simulink model "NAVI_V1"  (R2018a)
settings: configuration reference "Config_Ctrl" (kept outside this file)
PreLoadFcn:
  | NAVI_V1_BusInfo;
libraries: simulink x2
settings Model: Creator=IAEC nishito  LastModifiedBy=E00026
settings ConfigSetRef: SourceLocation=Base Workspace

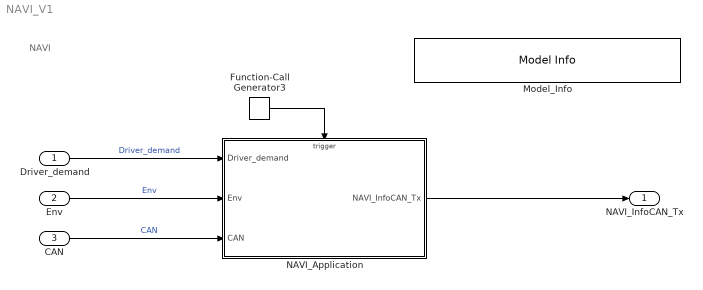
== system NAVI_V1 ==
  note: NAVI
  Driver_demand : Inport  OutDataTypeStr=Bus: Driver_demand_Bus
      settings: AttributesFormatString=<%<OutDataTypeStr>>
  Env : Inport  Port=2  OutDataTypeStr=Bus: Environment_Bus
      settings: AttributesFormatString=<%<OutDataTypeStr>>
  CAN : Inport  Port=3  OutDataTypeStr=Bus: CAN_Bus
      settings: AttributesFormatString=<%<OutDataTypeStr>>
  Function-Call Generator3 : simulink/Ports & Subsystems/Function-Call Generator  sample_time=0.1  numberOfIterations=1
      settings: AttributesFormatString=<sample_time=%<sample_time>>
  Model_Info : simulink/Model-Wide Utilities/Model Info  Frame=on  DisplayStringWithTags=|  HorizontalTextAlignment=Left  LeftAlignmentValue=0.02
      | Version  %<ModelVersion>
      | LastModifided by %<LastModifiedBy>  Date %<LastModificationDate>
      | Description  %<Description>
  NAVI_Application : Subsystem
  NAVI_InfoCAN_Tx : Outport  OutDataTypeStr=Bus: NAVI_InfoCAN_Tx_Bus
      settings: AttributesFormatString=<%<OutDataTypeStr>>
  wires:
  NAVI_Application/1(NAVI_InfoCAN_Tx) -> NAVI_InfoCAN_Tx/1
  CAN/1 -> NAVI_Application/3(CAN)  "CAN"
  Driver_demand/1 -> NAVI_Application/1(Driver_demand)  "Driver_demand"
  Function-Call Generator3/1 -> NAVI_Application/Trigger
  Env/1 -> NAVI_Application/2(Env)  "Env"

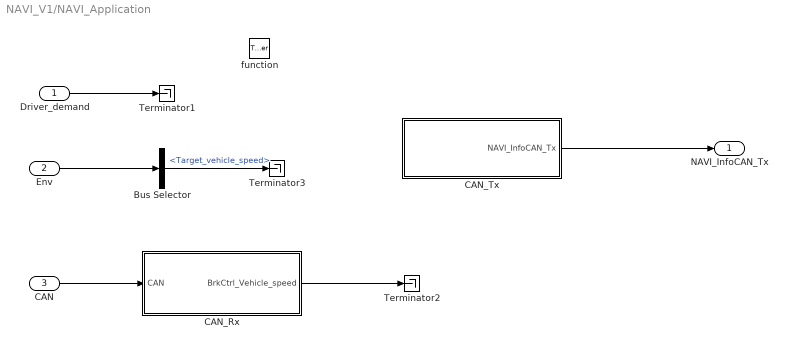
== system NAVI_V1/NAVI_Application ==
  Driver_demand : Inport
  Env : Inport  Port=2
  CAN : Inport  Port=3
  function : TriggerPort  TriggerType=function-call  VariantControl=Variant
  Bus Selector : BusSelector  OutputSignals=Target_vehicle_speed
  CAN_Rx : Subsystem
  CAN_Tx : Subsystem
  Terminator1 : Terminator
  Terminator2 : Terminator
  Terminator3 : Terminator
  NAVI_InfoCAN_Tx : Outport
  wires:
  Driver_demand/1 -> Terminator1/1
  CAN/1 -> CAN_Rx/1(CAN)
  CAN_Rx/1(BrkCtrl_Vehicle_speed) -> Terminator2/1
  Env/1 -> Bus Selector/1
  Bus Selector/1 -> Terminator3/1  "<Target_vehicle_speed>"
  CAN_Tx/1(NAVI_InfoCAN_Tx) -> NAVI_InfoCAN_Tx/1

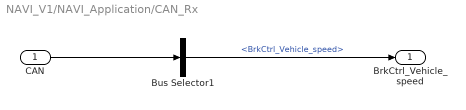
== system NAVI_V1/NAVI_Application/CAN_Rx ==
  CAN : Inport
  Bus Selector1 : BusSelector  OutputSignals=VehCAN.BrakeCtrl_VehCAN_Tx.BrkCtrl_Vehicle_speed
  BrkCtrl_Vehicle_speed : Outport
  wires:
  CAN/1 -> Bus Selector1/1
  Bus Selector1/1 -> BrkCtrl_Vehicle_speed/1  "<BrkCtrl_Vehicle_speed>"

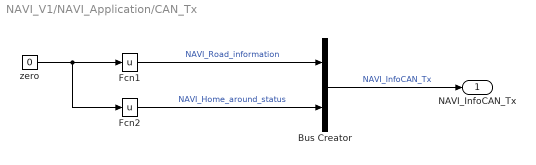
== system NAVI_V1/NAVI_Application/CAN_Tx ==
  Bus Creator : BusCreator  Inputs=2  OutDataTypeStr=Bus: NAVI_InfoCAN_Tx_Bus
      settings: AttributesFormatString=<%<OutDataTypeStr>>
  Fcn1 : Fcn  Expr=u
  Fcn2 : Fcn  Expr=u
  zero : Constant  Value=0
  NAVI_InfoCAN_Tx : Outport
  wires:
  Fcn1/1 -> Bus Creator/1  "NAVI_Road_information"
  zero/1 -> Fcn1/1, Fcn2/1
  Fcn2/1 -> Bus Creator/2  "NAVI_Home_around_status"
  Bus Creator/1 -> NAVI_InfoCAN_Tx/1  "NAVI_InfoCAN_Tx"
